simulink model "akh_rev_project"  (R2020b)
settings: Solver=ode45  StartTime=0.0  StopTime=10  FixedStep=Ts_Power  RelTol=1e-3  AbsTol=1e-2
InitFcn:
  | Fnom = 50;        % Hz
  | 
  | Fc = 27*Fnom;   % (Hz)
  | Ts_Power = 1/(Fc*100);
  | Ts_Control = Ts_Power*10;
values from neighbouring files (symbols this model uses):
  Ts = 1/fs    (= 1e-05)    [PE_46.m]    (also in disc_sim.m = 1; mass_spring_damper_model.m = 0.1)
undefined symbols (not defined in the file or in its folder): D1, D11, Delta, DiscIntNeverNeededParam, j, magnitude
libraries: powerlib x146, powerlib_meascontrol x90, simulink x2, re_lib x1
(part 5 of 8)

== system akh_rev_project/AC System 1/Wind Turbine Protection/Protection System/AC Current Protection ==
  abc : Inport  PortDimensions=3
  Complex to Magnitude-Angle1 : ComplexToMagnitudeAngle  Output=Magnitude
  Current Measurement : Subsystem
  MinMax : MinMax  Function=max  InputSameDT=on  SaturateOnIntegerOverflow=on  ZeroCross=off
  Mux : Mux  Inputs=3
  On Delay : powerlib_meascontrol/Logic/On Delay  DelayType=On delay  delay=Delay_I1  ic=0  Ts=0
  On Delay1 : powerlib_meascontrol/Logic/On Delay  DelayType=On delay  delay=Delay_I2_I1  ic=0  Ts=0
  Relational Operator10 : RelationalOperator  Operator=>  RndMeth=Nearest
  Relational Operator6 : RelationalOperator  Operator=>  RndMeth=Nearest
  Relational Operator8 : RelationalOperator  Operator=>  RndMeth=Nearest
  Selector : Selector  InputPortWidth=3  IndexOptions=Index vector (dialog)  Indices=1  OutputSizes=1
  Selector1 : Selector  InputPortWidth=3  IndexOptions=Index vector (dialog)  Indices=2  OutputSizes=1
  Selector2 : Selector  InputPortWidth=3  IndexOptions=Index vector (dialog)  Indices=3  OutputSizes=1
  V0/V1 max3 : Constant  Value=Max_I1
  V1 max : Constant  Value=Max_I2_I1
  V1 max2 : Constant  Value=Max_Iinst
  MaxIinst : Outport  VectorParamsAs1DForOutWhenUnconnected=off
  MaxI1 : Outport  Port=2  VectorParamsAs1DForOutWhenUnconnected=off
  MaxI2I1 : Outport  Port=3  VectorParamsAs1DForOutWhenUnconnected=off
  wires:
  abc/1 -> Current Measurement/1(abc), Selector/1, Selector1/1, Selector2/1
  Current Measurement/1(I1) -> Relational Operator6/1
  V0/V1 max3/1 -> Relational Operator6/2
  V1 max/1 -> Relational Operator8/2
  Current Measurement/2(I2/I1) -> Relational Operator8/1
  Relational Operator6/1 -> On Delay/1
  Relational Operator8/1 -> On Delay1/1
  On Delay/1 -> MaxI1/1
  On Delay1/1 -> MaxI2I1/1
  Relational Operator10/1 -> MaxIinst/1
  V1 max2/1 -> Relational Operator10/2
  Selector/1 -> Mux/1
  Selector2/1 -> Mux/3
  Selector1/1 -> Mux/2
  Mux/1 -> Complex to Magnitude-Angle1/1
  Complex to Magnitude-Angle1/1 -> MinMax/1
  MinMax/1 -> Relational Operator10/1

== system akh_rev_project/AC System 1/Wind Turbine Protection/Protection System/AC Voltage Protection ==
  abc : Inport  PortDimensions=3
  On Delay : powerlib_meascontrol/Logic/On Delay  DelayType=On delay  delay=Delay_V1  ic=0  Ts=0
  On Delay1 : powerlib_meascontrol/Logic/On Delay  DelayType=On delay  delay=Delay_V2_V1  ic=0  Ts=0
  On Delay2 : powerlib_meascontrol/Logic/On Delay  DelayType=On delay  delay=Delay_V1  ic=0  Ts=0
  On Delay3 : powerlib_meascontrol/Logic/On Delay  DelayType=On delay  delay=Delay_V2_V1  ic=0  Ts=0
  Relational Operator6 : RelationalOperator  Operator=>  RndMeth=Nearest
  Relational Operator7 : RelationalOperator  Operator=<  RndMeth=Nearest
  Relational Operator8 : RelationalOperator  Operator=>  RndMeth=Nearest
  Relational Operator9 : RelationalOperator  Operator=>  RndMeth=Nearest
  V0/V1 max3 : Constant  Value=Max_V1
  V0/V1 max4 : Constant  Value=Min_V1
  V1 max : Constant  Value=Max_V2_V1
  V1 max1 : Constant  Value=Max_V0_V1
  Voltage Measurement : Subsystem
  MinV1 : Outport  VectorParamsAs1DForOutWhenUnconnected=off
  MaxV1 : Outport  Port=2  VectorParamsAs1DForOutWhenUnconnected=off
  MaxV2V1 : Outport  Port=3  VectorParamsAs1DForOutWhenUnconnected=off
  MaxV0V1 : Outport  Port=4  VectorParamsAs1DForOutWhenUnconnected=off
  wires:
  On Delay3/1 -> MaxV0V1/1
  On Delay1/1 -> MaxV2V1/1
  On Delay/1 -> MinV1/1
  On Delay2/1 -> MaxV1/1
  Relational Operator9/1 -> On Delay3/1
  Relational Operator8/1 -> On Delay1/1
  Relational Operator7/1 -> On Delay/1
  Relational Operator6/1 -> On Delay2/1
  Voltage Measurement/3(V0/V1) -> Relational Operator9/1
  V1 max1/1 -> Relational Operator9/2
  Voltage Measurement/2(V2/V1) -> Relational Operator8/1
  V1 max/1 -> Relational Operator8/2
  V0/V1 max4/1 -> Relational Operator7/2
  V0/V1 max3/1 -> Relational Operator6/2
  Voltage Measurement/1(V1) -> Relational Operator7/1, Relational Operator6/1
  abc/1 -> Voltage Measurement/1(abc)

== system akh_rev_project/AC System 1/Wind Turbine Protection/Protection System/DC Voltage Protection ==
  Vdc : Inport
  On Delay : powerlib_meascontrol/Logic/On Delay  DelayType=On delay  delay=Delay_Vdc  ic=0  Ts=0
  Relational Operator1 : RelationalOperator  Operator=>  RndMeth=Nearest
  V1 max3 : Constant  Value=Max_Vdc
  MaxVdc : Outport  VectorParamsAs1DForOutWhenUnconnected=off
  wires:
  Vdc/1 -> Relational Operator1/1
  V1 max3/1 -> Relational Operator1/2
  Relational Operator1/1 -> On Delay/1
  On Delay/1 -> MaxVdc/1

== system akh_rev_project/AC System 1/Wind Turbine Protection/Protection System/Decoding ==
  Code : Inport
  Constant : Constant  Value=pow2(0:-1:-9)
  Constant6 : Constant  Value=2
  Math Function : Math  Operator=rem  SignedPower=on  SaturateOnIntegerOverflow=on
  Product : Product  InputSameDT=on  SaturateOnIntegerOverflow=on  OutDataTypeStr=Inherit: Same as first input
  Rounding Function : Rounding
  Out : Outport  VectorParamsAs1DForOutWhenUnconnected=off
  wires:
  Constant/1 -> Product/2
  Code/1 -> Product/1
  Product/1 -> Rounding Function/1
  Constant6/1 -> Math Function/2
  Rounding Function/1 -> Math Function/1
  Math Function/1 -> Out/1

== system akh_rev_project/AC System 1/Wind Turbine Protection/Protection System/Encoding ==
  In1 : Inport
  In2 : Inport  Port=2
  In3 : Inport  Port=3
  In4 : Inport  Port=4
  In5 : Inport  Port=5
  In6 : Inport  Port=6
  In7 : Inport  Port=7
  In8 : Inport  Port=8
  In9 : Inport  Port=9
  In10 : Inport  Port=10
  Constant12 : Constant  Value=pow2(0:1:9)
  Data Type Conversion : DataTypeConversion  SaturateOnIntegerOverflow=on  RndMeth=Zero
  Mux : Mux  Inputs=10
  Product : Product  InputSameDT=on  SaturateOnIntegerOverflow=on  OutDataTypeStr=Inherit: Same as first input
  Sum : Sum  Inputs=1  InputSameDT=on  SaturateOnIntegerOverflow=on  OutDataTypeStr=Inherit: Same as first input
  Code : Outport  VectorParamsAs1DForOutWhenUnconnected=off
  wires:
  Data Type Conversion/1 -> Product/1
  Mux/1 -> Data Type Conversion/1
  In2/1 -> Mux/2
  In3/1 -> Mux/3
  In4/1 -> Mux/4
  In5/1 -> Mux/5
  In6/1 -> Mux/6
  In7/1 -> Mux/7
  In8/1 -> Mux/8
  In9/1 -> Mux/9
  In10/1 -> Mux/10
  In1/1 -> Mux/1
  Product/1 -> Sum/1
  Constant12/1 -> Product/2
  Sum/1 -> Code/1

== system akh_rev_project/AC System 1/Wind Turbine Protection/Protection System/Sample & Hold ==
  note: Silvano Casoria
      | Power System Simulation Laboratory
      | IREQ, Hydro-Quebc
  note: Sample and Hold
  In : Inport
  S : Inport  Port=2
  IC=ic : Memory  InitialCondition=ic  InheritSampleTime=on
  Switch : Switch  Threshold=0.5  SaturateOnIntegerOverflow=on  InputSameDT=on
  "   " : Outport  InitialOutput=0  VectorParamsAs1DForOutWhenUnconnected=off
  wires:
  S/1 -> Switch/2
  In/1 -> Switch/1
  IC=ic/1 -> Switch/3
  Switch/1 -> IC=ic/1, "   "/1

== system akh_rev_project/AC System 1/Wind Turbine Protection/Protection System/Sample & Hold1 ==
  note: Silvano Casoria
      | Power System Simulation Laboratory
      | IREQ, Hydro-Quebc
  note: Sample and Hold
  In : Inport
  S : Inport  Port=2
  IC=ic : Memory  InitialCondition=ic  InheritSampleTime=on
  Switch : Switch  Threshold=0.5  SaturateOnIntegerOverflow=on  InputSameDT=on
  "   " : Outport  InitialOutput=0  VectorParamsAs1DForOutWhenUnconnected=off
  wires:
  S/1 -> Switch/2
  In/1 -> Switch/1
  IC=ic/1 -> Switch/3
  Switch/1 -> IC=ic/1, "   "/1

== system akh_rev_project/AC System 1/Wind Turbine Protection/Protection System/Under//Over Speed Protection ==
  Speed : Inport  PortDimensions=1
  On Delay : powerlib_meascontrol/Logic/On Delay  DelayType=On delay  delay=Delay_Speed  ic=0  Ts=0
  On Delay1 : powerlib_meascontrol/Logic/On Delay  DelayType=On delay  delay=Delay_Speed  ic=0  Ts=0
  Relational Operator1 : RelationalOperator  Operator=>  RndMeth=Nearest
  Relational Operator3 : RelationalOperator  Operator=<  RndMeth=Nearest
  V1 max1 : Constant  Value=Min_Speed
  V1 max3 : Constant  Value=Max_Speed
  MinSpeed : Outport  VectorParamsAs1DForOutWhenUnconnected=off
  MaxSpeed : Outport  Port=2  VectorParamsAs1DForOutWhenUnconnected=off
  wires:
  Relational Operator3/1 -> On Delay/1
  Relational Operator1/1 -> On Delay1/1
  V1 max1/1 -> Relational Operator3/2
  V1 max3/1 -> Relational Operator1/2
  Speed/1 -> Relational Operator3/1, Relational Operator1/1
  On Delay/1 -> MinSpeed/1
  On Delay1/1 -> MaxSpeed/1

== system akh_rev_project/VSC Controller Station 1/Discrete VSC Controller /Clark Transformations/CLARK  with Rotating reference ==
  note: Rotation of pi/6
  note: Rotation of - pi/6
  note: Reference rotation:
      | Type [0,1,2]          Rotation (rad)
      | 0                            0
      | 1                            - pi/6
      | 2                              pi/6
  note: CLARK transformations
  abc : Inport
  Type : Inport  Port=2
  CLARK : Subsystem  TreatAsAtomicUnit=on
  CLARK_lag : Subsystem  TreatAsAtomicUnit=on
  CLARK_lead : Subsystem  TreatAsAtomicUnit=on
  Constant : Constant  Value=2
  Constant1 : Constant  Value=0
  Constant2 : Constant
  Relational Operator1 : RelationalOperator  Operator===  RndMeth=Nearest  InputSameDT=on
  Relational Operator2 : RelationalOperator  Operator===  RndMeth=Nearest  InputSameDT=on
  Relational Operator3 : RelationalOperator  Operator===  RndMeth=Nearest  InputSameDT=on
  Sum : Sum  Inputs=+++  SaturateOnIntegerOverflow=on
  AB0 : Outport  VectorParamsAs1DForOutWhenUnconnected=off
  wires:
  Constant2/1 -> Relational Operator3/2
  Relational Operator2/1 -> CLARK/Enable
  Constant1/1 -> Relational Operator2/2
  CLARK/1(AB0) -> Sum/3
  Sum/1 -> AB0/1
  CLARK_lag/1(AB0) -> Sum/2
  CLARK_lead/1(AB0) -> Sum/1
  abc/1 -> CLARK/1(abc), CLARK_lag/1(abc), CLARK_lead/1(abc)
  Relational Operator1/1 -> CLARK_lead/Enable
  Relational Operator3/1 -> CLARK_lag/Enable
  Type/1 -> Relational Operator3/1, Relational Operator2/1, Relational Operator1/1
  Constant/1 -> Relational Operator1/2

== system akh_rev_project/VSC Controller Station 1/Discrete VSC Controller /Clark Transformations/CLARK  with Rotating reference1 ==
  note: Rotation of pi/6
  note: Rotation of - pi/6
  note: Reference rotation:
      | Type [0,1,2]          Rotation (rad)
      | 0                            0
      | 1                            - pi/6
      | 2                              pi/6
  note: CLARK transformations
  abc : Inport
  Type : Inport  Port=2
  CLARK : Subsystem  TreatAsAtomicUnit=on
  CLARK_lag : Subsystem  TreatAsAtomicUnit=on
  CLARK_lead : Subsystem  TreatAsAtomicUnit=on
  Constant : Constant  Value=2
  Constant1 : Constant  Value=0
  Constant2 : Constant
  Relational Operator1 : RelationalOperator  Operator===  RndMeth=Nearest  InputSameDT=on
  Relational Operator2 : RelationalOperator  Operator===  RndMeth=Nearest  InputSameDT=on
  Relational Operator3 : RelationalOperator  Operator===  RndMeth=Nearest  InputSameDT=on
  Sum : Sum  Inputs=+++  SaturateOnIntegerOverflow=on
  AB0 : Outport  VectorParamsAs1DForOutWhenUnconnected=off
  wires:
  Constant2/1 -> Relational Operator3/2
  Relational Operator2/1 -> CLARK/Enable
  Constant1/1 -> Relational Operator2/2
  CLARK/1(AB0) -> Sum/3
  Sum/1 -> AB0/1
  CLARK_lag/1(AB0) -> Sum/2
  CLARK_lead/1(AB0) -> Sum/1
  abc/1 -> CLARK/1(abc), CLARK_lag/1(abc), CLARK_lead/1(abc)
  Relational Operator1/1 -> CLARK_lead/Enable
  Relational Operator3/1 -> CLARK_lag/Enable
  Type/1 -> Relational Operator3/1, Relational Operator2/1, Relational Operator1/1
  Constant/1 -> Relational Operator1/2

== system akh_rev_project/VSC Controller Station 1/Discrete VSC Controller /DC Voltage Balance Control/Regulator ==
  note: Reset states when enabling
  note: Voltage Sign
  note: Reversed Current Sign
  V_ref_lim_abc : Inport
  Iv_abc : Inport  Port=2
  Udc_0_mean : Inport  Port=3
  Enable : EnablePort  StatesWhenEnabling=reset  PropagateVarSize=During execution
  Constant1 : Constant  Value=0
  Constant2 : Constant  Value=0
  Constant3 : Constant  Value=-1
  Constant4 : Constant
  Constant5 : Constant
  Constant6 : Constant  Value=-1
  Constant7 : Constant  Value=0
  PI_regulator (type 2) : Subsystem  mask(PI regulator with anti-windup - type 2){max_i=max_out_dcvbc, min_i=min_out_dcvbc, Ki=Ki_dcvbc, i_ic=0, Kp=Kp_dcvbc, Kf=1.0, max_out=max_out_dcvbc, min_out=min_out_dcvbc, Ts=Ts_Control}
      mask prompts: max_i "Integrator maximum  limit (pu):"; min_i "Integrator minimum  limit (pu):"; Ki "Integrator gain (pu/s):"; i_ic "Integrator initial condition (pu):"; Kp "Proportional gain:"; Kf "Feadback gain :"; max_out "Output maximum limit (pu):"; min_out "Output minimum limit (pu):"; Ts "Sample time: (s)"
      mask help:
      | The error signal (input 1 - input 2) is integrated with dynamic limits (Integrator min and max limits).
      | A back-calculation anti-windup method discharges the integrator on block saturation (output min and max limits) using a feedback loop having a gain coefficient.
      mask Display: disp('PI \n(Type 2)')
  Product : Product  Inputs=3  SaturateOnIntegerOverflow=on  OutDataTypeStr=Inherit: Same as first input
  Relational Operator : RelationalOperator  Operator=<  RndMeth=Nearest
  Relational Operator1 : RelationalOperator  Operator=<  RndMeth=Nearest
  Switch : Switch  Criteria=u2 > Threshold  SaturateOnIntegerOverflow=on
  Switch1 : Switch  Criteria=u2 > Threshold  SaturateOnIntegerOverflow=on
  dV_ref_abc_dcvbc : Outport  VectorParamsAs1DForOutWhenUnconnected=off
  wires:
  Constant1/1 -> PI_regulator (type 2)/2(Meas)
  Switch1/1 -> Product/2
  PI_regulator (type 2)/1(Out) -> Product/3
  Constant2/1 -> Relational Operator/2
  Constant3/1 -> Switch/1
  Constant4/1 -> Switch/3
  Relational Operator/1 -> Switch/2
  Constant5/1 -> Switch1/1
  Constant6/1 -> Switch1/3
  Relational Operator1/1 -> Switch1/2
  Switch/1 -> Product/1
  V_ref_lim_abc/1 -> Relational Operator/1
  Product/1 -> dV_ref_abc_dcvbc/1
  Iv_abc/1 -> Relational Operator1/1
  Udc_0_mean/1 -> PI_regulator (type 2)/1(Ord)
  Constant7/1 -> Relational Operator1/2

== system akh_rev_project/VSC Controller Station 1/Discrete VSC Controller /Inner Current Loop/AC_Current_Control ==
  note: Gain equal to the converter series reactance in pu
      | (ex: X transformer + X phase reactor)
  note: Uq
  note: Ud
  note: AC Current Control
  note: d axis
  note: q axis
  Iv_dq : Inport
  Iref_dq : Inport  Port=2
  U_dq : Inport  Port=3
  Freq : Inport  Port=4
  Demux : Demux  Outputs=2
      settings: DisplayOption=none
  Demux1 : Demux  Outputs=2
      settings: DisplayOption=none
  Demux2 : Demux  Outputs=2
      settings: DisplayOption=none
  Gain : Gain  Gain=Kf_accc
  Gain1 : Gain  Gain=Kf_accc
  "Mean (Variable Frequency, IC=1)" : powerlib_meascontrol/Measurements/Mean (Variable Frequency)  Finit=Fnom  Fmin=f_min_pll  Vinit=1.0  Ts=Ts_Control
      settings: SourceProductBaseCode=PS
  "Mean (Variable Frequency, IC=1)  " : powerlib_meascontrol/Measurements/Mean (Variable Frequency)  Finit=Fnom  Fmin=f_min_pll  Vinit=1.0  Ts=Ts_Control
      settings: SourceProductBaseCode=PS
  Mux : Mux  Inputs=2
  PI_regulator 1 : Subsystem  mask(PI regulator with anti-windup - type 2){max_i=max_out_accc, min_i=min_out_accc, Ki=Ki_accc, i_ic=0, Kp=Kp_accc, Kf=1.0, max_out=max_out_accc, min_out=min_out_accc, Ts=Ts_Control}
      mask prompts: max_i "Integrator maximum  limit (pu):"; min_i "Integrator minimum  limit (pu):"; Ki "Integrator gain (pu/s):"; i_ic "Integrator initial condition (pu):"; Kp "Proportional gain:"; Kf "Feadback gain :"; max_out "Output maximum limit (pu):"; min_out "Output minimum limit (pu):"; Ts "Sample time: (s)"
      mask help:
      | The error signal (input 1 - input 2) is integrated with dynamic limits (Integrator min and max limits).
      | A back-calculation anti-windup method discharges the integrator on block saturation (output min and max limits) using a feedback loop having a gain coefficient.
      mask Display: disp('PI \n(Type 2)')
  PI_regulator 2 : Subsystem  mask(PI regulator with anti-windup - type 2){max_i=max_out_accc, min_i=min_out_accc, Ki=Ki_accc, i_ic=0, Kp=Kp_accc, Kf=1.0, max_out=max_out_accc, min_out=min_out_accc, Ts=Ts_Control}
      mask prompts: max_i "Integrator maximum  limit (pu):"; min_i "Integrator minimum  limit (pu):"; Ki "Integrator gain (pu/s):"; i_ic "Integrator initial condition (pu):"; Kp "Proportional gain:"; Kf "Feadback gain :"; max_out "Output maximum limit (pu):"; min_out "Output minimum limit (pu):"; Ts "Sample time: (s)"
      mask help:
      | The error signal (input 1 - input 2) is integrated with dynamic limits (Integrator min and max limits).
      | A back-calculation anti-windup method discharges the integrator on block saturation (output min and max limits) using a feedback loop having a gain coefficient.
      mask Display: disp('PI \n(Type 2)')
  Sum2 : Sum  Inputs=+|-|+  InputSameDT=on  SaturateOnIntegerOverflow=on  OutDataTypeStr=Inherit: Same as first input
  Sum3 : Sum  Inputs=--+  InputSameDT=on  SaturateOnIntegerOverflow=on  OutDataTypeStr=Inherit: Same as first input
  Vref_dq_tmp : Outport  VectorParamsAs1DForOutWhenUnconnected=off
  wires:
  PI_regulator 2/1(Out) -> Sum3/1
  Sum3/1 -> Mux/2
  "Mean (Variable Frequency, IC=1)  "/1 -> Sum3/3
  Demux2/2 -> "Mean (Variable Frequency, IC=1)  "/2
  Gain1/1 -> Sum3/2
  Sum2/1 -> Mux/1
  "Mean (Variable Frequency, IC=1)"/1 -> Sum2/1
  Freq/1 -> "Mean (Variable Frequency, IC=1)"/1, "Mean (Variable Frequency, IC=1)  "/1
  Demux2/1 -> "Mean (Variable Frequency, IC=1)"/2
  PI_regulator 1/1(Out) -> Sum2/2
  Iref_dq/1 -> Demux1/1
  Iv_dq/1 -> Demux/1
  Demux1/1 -> PI_regulator 1/1(Ord), Gain1/1  "I_ref_d"
  Demux/1 -> PI_regulator 1/2(Meas)  "Iv_d"
  Demux/2 -> PI_regulator 2/2(Meas)  "Iv_q"
  Mux/1 -> Vref_dq_tmp/1
  U_dq/1 -> Demux2/1
  Demux1/2 -> PI_regulator 2/1(Ord), Gain/1  "I_ref_q"
  Gain/1 -> Sum2/3

== system akh_rev_project/VSC Controller Station 1/Discrete VSC Controller /Inner Current Loop/Reference_Voltage_Conditioning ==
  note: Maximum AC Voltage / DC Voltage (pole-neutral)
  note: Voltage Reference Conditioning
  Vref_dq_tmp : Inport
  Udc_meas_mean : Inport  Port=2
  Constant2 : Constant  Value=K_pwm
  Gain1 : Gain  Gain=k_pu2nom_Vdc  SaturateOnIntegerOverflow=on  OutDataTypeStr=Inherit: Same as input  ParamDataTypeStr=Inherit: Same as input
  Product1 : Product  Inputs=**/  SaturateOnIntegerOverflow=on  OutDataTypeStr=Inherit: Same as first input
  Vref_dq : Outport  VectorParamsAs1DForOutWhenUnconnected=off
  wires:
  Gain1/1 -> Product1/2
  Udc_meas_mean/1 -> Gain1/1
  Product1/1 -> Vref_dq/1
  Vref_dq_tmp/1 -> Product1/1
  Constant2/1 -> Product1/3

== system akh_rev_project/VSC Controller Station 1/Discrete VSC Controller /Inner Current Loop/Reference_Voltage_Limitation ==
  note: Limitation on a circle of 1 p.u. radius
  note: Reference Voltage Limitation
  note: Not Limited
  note: Limited
  Vref_dq : Inport
  Constant2 : Constant  Value=1.0
  Math Function : Math  Operator=magnitude^2  SignedPower=on  SaturateOnIntegerOverflow=on
  Math Function1 : Math  Operator=sqrt  SignedPower=on  SaturateOnIntegerOverflow=on
  Max=inf Min=eps : Saturate  UpperLimit=1e6  LowerLimit=1e-6
  Product : Product  Inputs=/*  SaturateOnIntegerOverflow=on  OutDataTypeStr=Inherit: Same as first input
  Relational Operator1 : RelationalOperator  Operator=<  RndMeth=Nearest
  Sum : Sum  Inputs=+  SaturateOnIntegerOverflow=on
  Switch : Switch  Criteria=u2 > Threshold  SaturateOnIntegerOverflow=on
  Vref_lim_dq : Outport  VectorParamsAs1DForOutWhenUnconnected=off
  wires:
  Max=inf Min=eps/1 -> Product/1
  Relational Operator1/1 -> Switch/2
  Math Function1/1 -> Max=inf Min=eps/1, Relational Operator1/1
  Vref_dq/1 -> Math Function/1, Switch/1, Product/2
  Math Function/1 -> Sum/1
  Sum/1 -> Math Function1/1
  Product/1 -> Switch/3
  Switch/1 -> Vref_lim_dq/1
  Constant2/1 -> Relational Operator1/2

== system akh_rev_project/VSC Controller Station 1/Discrete VSC Controller /Outer Active-Reactive Power and Voltage Loop/Active_Power_Control ==
  note: Output is added to the regulator reference
      |  in order to maintain the DC voltage within
      |  minimum and maximum limits
  note: Active Power Control
  enable_control : Inport
  enable_ramp : Inport  Port=2
  Pref : Inport  Port=3
  dPref : Inport  Port=4
  P_meas : Inport  Port=5
  U_meas : Inport  Port=6
  Udc_meas : Inport  Port=7
  Add : Sum
  DC Voltage Control Override : Subsystem  mask(Regulator with override functionality){max_in=Udc_max, min_in=Udc_min, Ki=Ki_apc_vco, Kp=Kp_apc_vco, IC_i=0, max_out_lim=max_apc_vco, min_out_lim=min_apc_vco, Ts=Ts_Control}
      mask prompts: max_in "Input upper range (pu):"; min_in "Input lower range (pu):"; Ki "Integrator gain (pu/s):"; Kp "Proportional gain:"; IC_i "Integrator initial condition (pu):"; max_out_lim "Output maximum limit (pu):"; min_out_lim "Output minimum limit (pu):"; Ts "Sample time: (s)"
      mask Display: disp('Override \nRegulator')
  Freeze_integrator : Subsystem
  Int_regulator (type 1) : Subsystem  mask(Feed forward integral regulator with anti-windup and freeze - type 1){max_i=max_i_apc, min_i=min_i_apc, Ki=Ki_apc, IC_i=0, Kf=1.0, max_out=P_max, min_out=P_min, Ts=Ts_Control}
      mask prompts: max_i "Integrator maximum  limit (pu):"; min_i "Integrator minimum  limit (pu):"; Ki "Integrator gain (pu/s):"; IC_i "Integrator initial condition (pu):"; Kf "Feadback gain :"; max_out "Output maximum limit (pu):"; min_out "Output minimum limit (pu):"; Ts "Sample time: (s)"
      mask help:
      | The reference (input 1) is fed forward to the output. The integrator compensates for any steady-state error between the desired (input 1) and the measured value input 2). The error signal (input 1 - input 2) is integrated with dynamic limits (Integrator min and max limits). The integration can be frozen (stopped) when input 3 is TRUE.
      | A back-calculation anti-windup method discharges the integrator on block saturation (output min and max limits) using a feedback loop having a gain coefficient.
      mask Display: disp('Integral \n(Type 1)')
  Ramping : Subsystem
  Saturation : Saturate  UpperLimit=P_max  LowerLimit=P_min
      settings: AttributesFormatString=Min=%<LowerLimit>\nMax=%<UpperLimit>
  Sum2 : Sum  SaturateOnIntegerOverflow=on
  Pref_apc : Outport  VectorParamsAs1DForOutWhenUnconnected=off
  Pref_ramped : Outport  Port=2  VectorParamsAs1DForOutWhenUnconnected=off
  wires:
  DC Voltage Control Override/1(Out) -> Add/2
  Int_regulator (type 1)/1(Out) -> Add/1
  Freeze_integrator/1(Freeze) -> Int_regulator (type 1)/3(freeze)
  Add/1 -> Saturation/1
  Saturation/1 -> Pref_apc/1
  Udc_meas/1 -> DC Voltage Control Override/1(In)
  U_meas/1 -> Freeze_integrator/1(U_meas)
  enable_ramp/1 -> Ramping/1(enable_ramp)
  Pref/1 -> Ramping/2(Pref)
  P_meas/1 -> Int_regulator (type 1)/2(Meas)
  Sum2/1 -> Pref_ramped/1, Int_regulator (type 1)/1(Ord)
  dPref/1 -> Sum2/2
  Ramping/1(Pref_ramp) -> Sum2/1
  enable_control/1 -> Int_regulator (type 1)/Enable, DC Voltage Control Override/Enable

== system akh_rev_project/VSC Controller Station 1/Discrete VSC Controller /Outer Active-Reactive Power and Voltage Loop/Current_Reference_Calculation ==
  note: Current Reference Calculation
  Pref_apc : Inport
  Qref_rpc : Inport  Port=2
  Uf_meas : Inport  Port=3
  Constant24 : Constant  Value=U_level_crc
  MinMax : MinMax  Function=max  Inputs=2  InputSameDT=on  SaturateOnIntegerOverflow=on
  Product : Product  Inputs=*/  SaturateOnIntegerOverflow=on  OutDataTypeStr=Inherit: Same as first input
  Product1 : Product  Inputs=/*  SaturateOnIntegerOverflow=on  OutDataTypeStr=Inherit: Same as first input
  Saturation : Saturate  UpperLimit=lim_d_crc  LowerLimit=-lim_d_crc
      settings: AttributesFormatString=Min: %<LowerLimit>\nMax: %<UpperLimit>
  Saturation1 : Saturate  UpperLimit=lim_q_crc  LowerLimit=-lim_q_crc
      settings: AttributesFormatString=Min: %<LowerLimit>\nMax: %<UpperLimit>
  Saturation2 : Saturate  UpperLimit=inf  LowerLimit=eps
      settings: AttributesFormatString=Min: %<LowerLimit>\nMax: %<UpperLimit>
  Second-Order LP Filter : powerlib_meascontrol/Filters/Second-Order Filter  FilterType=Lowpass  Fo=f0_crc  Zeta=1/sqrt(2)  Ts=Ts_Control  Initialize=off  Vac_Init="[0,  0,  60]"  Vdc_Init=0  PlotResponse=off  FreqRange=[0, 500, 1]
      settings: AttributesFormatString=Fo: %<Fo>  SourceProductBaseCode=PS
  Iref_d_crc : Outport  VectorParamsAs1DForOutWhenUnconnected=off
  Iref_q_crc : Outport  Port=2  VectorParamsAs1DForOutWhenUnconnected=off
  wires:
  Second-Order LP Filter/1 -> MinMax/2
  Saturation1/1 -> Iref_q_crc/1
  Saturation/1 -> Iref_d_crc/1
  Uf_meas/1 -> Second-Order LP Filter/1
  Constant24/1 -> MinMax/1
  Pref_apc/1 -> Product/1
  Saturation2/1 -> Product/2, Product1/1
  Qref_rpc/1 -> Product1/2
  Product/1 -> Saturation/1
  Product1/1 -> Saturation1/1
  MinMax/1 -> Saturation2/1

== system akh_rev_project/VSC Controller Station 1/Discrete VSC Controller /Outer Active-Reactive Power and Voltage Loop/Current_Reference_Limitation ==
  note: DC Voltage Control mode (Active power priority)
  note: Power Control mode (Equal scaling)
  note: Current Reference Limitation
  Iref_d_tmp : Inport  PortDimensions=1
  Iref_q_tmp : Inport  Port=2  PortDimensions=1
  P_control : Inport  Port=3
  Constant25 : Constant  Value=Iref_max
  Double click here for  info : Subsystem
      mask Display: disp('?')
  Math Function1 : Math  Operator=sqrt  SignedPower=on  SaturateOnIntegerOverflow=on
  Math Function2 : Math  Operator=magnitude^2  SignedPower=on  SaturateOnIntegerOverflow=on
  Math Function3 : Math  Operator=magnitude^2  SignedPower=on  SaturateOnIntegerOverflow=on
  Math Function4 : Math  Operator=magnitude^2  SignedPower=on  SaturateOnIntegerOverflow=on
  Math Function5 : Math  Operator=sqrt  SignedPower=on  SaturateOnIntegerOverflow=on
  Min:eps Max:inf : Saturate  UpperLimit=1e6  LowerLimit=1e-6
  Mux : Mux  Inputs=2
  Mux1 : Mux  Inputs=2
  Product1 : Product  SaturateOnIntegerOverflow=on  OutDataTypeStr=Inherit: Same as first input
  Product2 : Product  Inputs=*/  SaturateOnIntegerOverflow=on  OutDataTypeStr=Inherit: Same as first input
  Relational Operator1 : RelationalOperator  RndMeth=Nearest
  Relational Operator3 : RelationalOperator  RndMeth=Nearest
  Sign : Signum
  Sum : Sum  Inputs=+  SaturateOnIntegerOverflow=on
  Sum2 : Sum  Inputs=-+  SaturateOnIntegerOverflow=on
  Switch1 : Switch  Criteria=u2 > Threshold  SaturateOnIntegerOverflow=on
  Switch2 : Switch  Criteria=u2 > Threshold  SaturateOnIntegerOverflow=on
  Switch3 : Switch  Criteria=u2 > Threshold  SaturateOnIntegerOverflow=on
  Iref_dq : Outport  VectorParamsAs1DForOutWhenUnconnected=off
  wires:
  Sign/1 -> Product1/2
  Math Function5/1 -> Product1/1
  Product1/1 -> Mux1/2
  Sum2/1 -> Math Function5/1
  Math Function4/1 -> Sum2/1
  Math Function3/1 -> Sum2/2
  Mux1/1 -> Switch2/3
  Switch1/1 -> Iref_dq/1
  Switch2/1 -> Switch1/1
  Product2/1 -> Switch2/1
  Min:eps Max:inf/1 -> Product2/2
  Relational Operator1/1 -> Switch1/2
  Constant25/1 -> Relational Operator3/2, Switch3/1, Math Function3/1, Relational Operator1/2
  Math Function1/1 -> Min:eps Max:inf/1, Relational Operator1/1
  Mux/1 -> Product2/1, Math Function2/1, Switch1/3
  Iref_q_tmp/1 -> Sign/1, Mux/2
  Iref_d_tmp/1 -> Relational Operator3/1, Switch3/3, Mux/1
  Sum/1 -> Math Function1/1
  Math Function2/1 -> Sum/1
  P_control/1 -> Switch2/2
  Relational Operator3/1 -> Switch3/2
  Switch3/1 -> Mux1/1, Math Function4/1

== system akh_rev_project/VSC Controller Station 1/Discrete VSC Controller /Outer Active-Reactive Power and Voltage Loop/DC_Voltage_Control ==
  note: DC Voltage Control
  note: Reset integrator when enabling
  Udref : Inport
  Udc_meas : Inport  Port=2
  Enable (Reset) : EnablePort  StatesWhenEnabling=reset  PropagateVarSize=During execution
  PI_regulator (type 2) : Subsystem  mask(PI regulator with anti-windup - type 2){max_i=max_i_dcvc, min_i=min_i_dcvc, Ki=Ki_dcvc, i_ic=0, Kp=Kp_dcvc, Kf=1.0, max_out=max_out_dcvc, min_out=min_out_dcvc, Ts=Ts_Control}
      mask prompts: max_i "Integrator maximum  limit (pu):"; min_i "Integrator minimum  limit (pu):"; Ki "Integrator gain (pu/s):"; i_ic "Integrator initial condition (pu):"; Kp "Proportional gain:"; Kf "Feadback gain :"; max_out "Output maximum limit (pu):"; min_out "Output minimum limit (pu):"; Ts "Sample time: (s)"
      mask help:
      | The error signal (input 1 - input 2) is integrated with dynamic limits (Integrator min and max limits).
      | A back-calculation anti-windup method discharges the integrator on block saturation (output min and max limits) using a feedback loop having a gain coefficient.
      mask Display: disp('PI \n(Type 2)')
  Iref_d_dcvc : Outport  VectorParamsAs1DForOutWhenUnconnected=off
  wires:
  PI_regulator (type 2)/1(Out) -> Iref_d_dcvc/1
  Udref/1 -> PI_regulator (type 2)/1(Ord)
  Udc_meas/1 -> PI_regulator (type 2)/2(Meas)

== system akh_rev_project/VSC Controller Station 1/Discrete VSC Controller /Outer Active-Reactive Power and Voltage Loop/Reactive_Power_Control ==
  note: Output is added to the regulator reference
      |  in order to maintain the AC voltage within
      |  minimum and maximum limits
  note: Reactive Power Control
  enable_control : Inport
  Qref : Inport  Port=2
  Q_meas : Inport  Port=3
  U_meas : Inport  Port=4
  "AC Voltage Control Override " : Subsystem  mask(Regulator with override functionality){max_in=U_max, min_in=U_min, Ki=Ki_rpc_vco, Kp=Kp_rpc_vco, IC_i=0, max_out_lim=max_rpc_vco, min_out_lim=min_rpc_vco, Ts=Ts_Control}
      mask prompts: max_in "Input upper range (pu):"; min_in "Input lower range (pu):"; Ki "Integrator gain (pu/s):"; Kp "Proportional gain:"; IC_i "Integrator initial condition (pu):"; max_out_lim "Output maximum limit (pu):"; min_out_lim "Output minimum limit (pu):"; Ts "Sample time: (s)"
      mask Display: disp('Override \nRegulator')
  Add : Sum
  Freeze_integrator : Subsystem
  Gain : Gain  Gain=-1
  Int_regulator (type 1) : Subsystem  mask(Feed forward integral regulator with anti-windup and freeze - type 1){max_i=max_i_rpc, min_i=min_i_rpc, Ki=Ki_rpc, IC_i=0, Kf=1.0, max_out=Q_max, min_out=Q_min, Ts=Ts_Control}
      mask prompts: max_i "Integrator maximum  limit (pu):"; min_i "Integrator minimum  limit (pu):"; Ki "Integrator gain (pu/s):"; IC_i "Integrator initial condition (pu):"; Kf "Feadback gain :"; max_out "Output maximum limit (pu):"; min_out "Output minimum limit (pu):"; Ts "Sample time: (s)"
      mask help:
      | The reference (input 1) is fed forward to the output. The integrator compensates for any steady-state error between the desired (input 1) and the measured value input 2). The error signal (input 1 - input 2) is integrated with dynamic limits (Integrator min and max limits). The integration can be frozen (stopped) when input 3 is TRUE.
      | A back-calculation anti-windup method discharges the integrator on block saturation (output min and max limits) using a feedback loop having a gain coefficient.
      mask Display: disp('Integral \n(Type 1)')
  Saturation : Saturate  UpperLimit=Q_max  LowerLimit=Q_min
      settings: AttributesFormatString=Min=%<LowerLimit>\nMax=%<UpperLimit>
  Qref_rpc : Outport  VectorParamsAs1DForOutWhenUnconnected=off
  wires:
  Gain/1 -> Add/1
  Add/1 -> Saturation/1
  "AC Voltage Control Override "/1(Out) -> Add/2
  Int_regulator (type 1)/1(Out) -> Gain/1
  U_meas/1 -> Freeze_integrator/1(U_meas), "AC Voltage Control Override "/1(In)
  Saturation/1 -> Qref_rpc/1
  Qref/1 -> Int_regulator (type 1)/1(Ord)
  Q_meas/1 -> Int_regulator (type 1)/2(Meas)
  enable_control/1 -> Int_regulator (type 1)/Enable, "AC Voltage Control Override "/Enable
  Freeze_integrator/1(Freeze) -> Int_regulator (type 1)/3(freeze)

== system akh_rev_project/VSC Controller Station 1/Discrete VSC Controller /PLL/Discrete PI Controller ==
  note: Pierre Giroux, Gilbert Sybille
      | Power System Simulation Laboratory
      | IREQ, Hydro-Quebc
  note: Discrete PID Controller
  Error : Inport  SampleTime=Ts
  Discrete-Time Integrator : DiscreteIntegrator  InitialCondition=Init  SampleTime=Ts  LimitOutput=on  UpperSaturationLimit=UpperLimit  LowerSaturationLimit=LowerLimit  ICPrevOutput=DiscIntNeverNeededParam  ICPrevScaledInput=DiscIntNeverNeededParam
  Kp4 : Gain  Gain=Kp  SaturateOnIntegerOverflow=on  SampleTime=Ts  OutDataTypeStr=Inherit: Same as input  ParamDataTypeStr=Inherit: Same as input
  Kp5 : Gain  Gain=Ki  SaturateOnIntegerOverflow=on  SampleTime=Ts  OutDataTypeStr=Inherit: Same as input  ParamDataTypeStr=Inherit: Same as input
  Saturation2 : Saturate  UpperLimit=UpperLimit  LowerLimit=LowerLimit  SampleTime=Ts
  Sum6 : Sum  InputSameDT=on  SaturateOnIntegerOverflow=on  SampleTime=Ts  OutDataTypeStr=Inherit: Same as first input
  Zero-Order Hold : ZeroOrderHold  SampleTime=Ts
  Out : Outport  SampleTime=Ts  InitialOutput=0  VectorParamsAs1DForOutWhenUnconnected=off
  wires:
  Error/1 -> Kp4/1, Kp5/1
  Sum6/1 -> Saturation2/1
  Kp5/1 -> Discrete-Time Integrator/1
  Kp4/1 -> Zero-Order Hold/1
  Discrete-Time Integrator/1 -> Sum6/2
  Saturation2/1 -> Out/1
  Zero-Order Hold/1 -> Sum6/1

== system akh_rev_project/VSC Controller Station 1/Discrete VSC Controller /PLL/Discrete Rate Limiter ==
  note: Delta(u)
  note: Beat Ronner
      | ABB Industrie AG
      | Turgi, Switzerland
  In : Inport
  Saturation : Saturate  UpperLimit=UpperLimit  LowerLimit=LowerLimit
  Sum : Sum  Inputs=|++  InputSameDT=on  SaturateOnIntegerOverflow=on  OutDataTypeStr=Inherit: Same as first input
  Sum1 : Sum  Inputs=|+-  InputSameDT=on  SaturateOnIntegerOverflow=on  OutDataTypeStr=Inherit: Same as first input
  Unit Delay : UnitDelay  InitialCondition=Vinit  SampleTime=Ts  HasFrameUpgradeWarning=on
  Out : Outport  VectorParamsAs1DForOutWhenUnconnected=off
  wires:
  In/1 -> Sum1/1  "u"
  Sum1/1 -> Saturation/1
  Saturation/1 -> Sum/1  "Delta(u)_limit"
  Sum/1 -> Out/1, Unit Delay/1  "y"
  Unit Delay/1 -> Sum1/2, Sum/2  "y-1"

== system akh_rev_project/VSC Controller Station 1/Discrete VSC Controller /Signal Calculations/Active_Power ==
  note: Active Power Calculation
  U_AB : Inport
  I_AB : Inport  Port=2
  Demux : Demux  Outputs=2
      settings: DisplayOption=none
  Demux1 : Demux  Outputs=2
      settings: DisplayOption=none
  Product : Product  SaturateOnIntegerOverflow=on  OutDataTypeStr=Inherit: Same as first input
  Product1 : Product  SaturateOnIntegerOverflow=on  OutDataTypeStr=Inherit: Same as first input
  Sum : Sum  SaturateOnIntegerOverflow=on
  Ppcc : Outport  VectorParamsAs1DForOutWhenUnconnected=off
  wires:
  U_AB/1 -> Demux/1
  I_AB/1 -> Demux1/1
  Demux/1 -> Product/1
  Demux1/1 -> Product/2
  Demux/2 -> Product1/1
  Demux1/2 -> Product1/2
  Product/1 -> Sum/1
  Product1/1 -> Sum/2
  Sum/1 -> Ppcc/1

== system akh_rev_project/VSC Controller Station 1/Discrete VSC Controller /Signal Calculations/DC_Current ==
  note: DC Current Calculation
  Idc_p : Inport
  Idc_n : Inport  Port=2
  Gain : Gain  Gain=0.5  SaturateOnIntegerOverflow=on  OutDataTypeStr=Inherit: Same as input  ParamDataTypeStr=Inherit: Same as input
  Sum : Sum  Inputs=+-  SaturateOnIntegerOverflow=on
  Idc_meas : Outport  VectorParamsAs1DForOutWhenUnconnected=off
  wires:
  Gain/1 -> Idc_meas/1
  Sum/1 -> Gain/1
  Idc_n/1 -> Sum/2
  Idc_p/1 -> Sum/1

== system akh_rev_project/VSC Controller Station 1/Discrete VSC Controller /Signal Calculations/DC_Voltage ==
  note: DC Voltage Calculation
  Udc_p : Inport
  Udc_n : Inport  Port=2
  Gain : Gain  Gain=0.5  SaturateOnIntegerOverflow=on  OutDataTypeStr=Inherit: Same as input  ParamDataTypeStr=Inherit: Same as input
  Sum : Sum  Inputs=+-  SaturateOnIntegerOverflow=on
  Udc_meas : Outport  VectorParamsAs1DForOutWhenUnconnected=off
  wires:
  Udc_p/1 -> Sum/1
  Sum/1 -> Gain/1
  Gain/1 -> Udc_meas/1
  Udc_n/1 -> Sum/2

== system akh_rev_project/VSC Controller Station 1/Discrete VSC Controller /Signal Calculations/Filter_Bus_Voltage ==
  note: Filter Bus Voltage Calculation
  Uf_AB : Inport
  Math Function : Math  Operator=magnitude^2  SignedPower=on  SaturateOnIntegerOverflow=on
  Math Function1 : Math  Operator=sqrt  SignedPower=on  SaturateOnIntegerOverflow=on
  Sum : Sum  Inputs=+  SaturateOnIntegerOverflow=on
  Uf_meas : Outport  VectorParamsAs1DForOutWhenUnconnected=off
  wires:
  Math Function1/1 -> Uf_meas/1
  Sum/1 -> Math Function1/1
  Math Function/1 -> Sum/1
  Uf_AB/1 -> Math Function/1

== system akh_rev_project/VSC Controller Station 1/Discrete VSC Controller /Signal Calculations/Modulation_Index ==
  note: Modulation Index Calculation
  Vref_lim_AB : Inport
  Udc_meas : Inport  Port=2
  Gain1 : Gain  Gain=k_pu2nom_Vdc  SaturateOnIntegerOverflow=on  OutDataTypeStr=Inherit: Same as input  ParamDataTypeStr=Inherit: Same as input
  MAX:10 MIN: 0 : Saturate  UpperLimit=10  LowerLimit=0
  Math Function1 : Math  Operator=magnitude^2  SignedPower=on  SaturateOnIntegerOverflow=on
  Math Function2 : Math  Operator=sqrt  SignedPower=on  SaturateOnIntegerOverflow=on
  Product : Product  Inputs=*/  SaturateOnIntegerOverflow=on  OutDataTypeStr=Inherit: Same as first input
  Saturation : Saturate  UpperLimit=1e6  LowerLimit=1e-6
  Sum : Sum  Inputs=+  SaturateOnIntegerOverflow=on
  Mod_index : Outport  VectorParamsAs1DForOutWhenUnconnected=off
  wires:
  Gain1/1 -> Saturation/1
  MAX:10 MIN: 0/1 -> Mod_index/1
  Saturation/1 -> Product/2
  Product/1 -> MAX:10 MIN: 0/1
  Udc_meas/1 -> Gain1/1
  Sum/1 -> Math Function2/1
  Math Function1/1 -> Sum/1
  Math Function2/1 -> Product/1
  Vref_lim_AB/1 -> Math Function1/1

== system akh_rev_project/VSC Controller Station 1/Discrete VSC Controller /Signal Calculations/PCC_Voltage ==
  note: Active Power Calculation
  U_AB : Inport
  Math Function : Math  Operator=magnitude^2  SignedPower=on  SaturateOnIntegerOverflow=on
  Math Function1 : Math  Operator=sqrt  SignedPower=on  SaturateOnIntegerOverflow=on
  Sum : Sum  Inputs=+  SaturateOnIntegerOverflow=on
  Upcc : Outport  VectorParamsAs1DForOutWhenUnconnected=off
  wires:
  U_AB/1 -> Math Function/1
  Math Function/1 -> Sum/1
  Sum/1 -> Math Function1/1
  Math Function1/1 -> Upcc/1

== system akh_rev_project/VSC Controller Station 1/Discrete VSC Controller /Signal Calculations/Reactive_Power ==
  note: Reactive Power Calculation
  U_AB : Inport
  I_AB : Inport  Port=2
  Demux : Demux  Outputs=2
      settings: DisplayOption=none
  Demux1 : Demux  Outputs=2
      settings: DisplayOption=none
  Product : Product  SaturateOnIntegerOverflow=on  OutDataTypeStr=Inherit: Same as first input
  Product1 : Product  SaturateOnIntegerOverflow=on  OutDataTypeStr=Inherit: Same as first input
  Sum : Sum  Inputs=+-  SaturateOnIntegerOverflow=on
  Qpcc : Outport  VectorParamsAs1DForOutWhenUnconnected=off
  wires:
  Sum/1 -> Qpcc/1
  Product1/1 -> Sum/2
  Product/1 -> Sum/1
  I_AB/1 -> Demux1/1
  U_AB/1 -> Demux/1
  Demux/2 -> Product/2
  Demux1/1 -> Product/1
  Demux/1 -> Product1/1
  Demux1/2 -> Product1/2

== system akh_rev_project/VSC Controller Station 2/Discrete VSC Controller /Clark Transformations/CLARK  with Rotating reference ==
  note: Rotation of pi/6
  note: Rotation of - pi/6
  note: Reference rotation:
      | Type [0,1,2]          Rotation (rad)
      | 0                            0
      | 1                            - pi/6
      | 2                              pi/6
  note: CLARK transformations
  abc : Inport
  Type : Inport  Port=2
  CLARK : Subsystem  TreatAsAtomicUnit=on
  CLARK_lag : Subsystem  TreatAsAtomicUnit=on
  CLARK_lead : Subsystem  TreatAsAtomicUnit=on
  Constant : Constant  Value=2
  Constant1 : Constant  Value=0
  Constant2 : Constant
  Relational Operator1 : RelationalOperator  Operator===  RndMeth=Nearest  InputSameDT=on
  Relational Operator2 : RelationalOperator  Operator===  RndMeth=Nearest  InputSameDT=on
  Relational Operator3 : RelationalOperator  Operator===  RndMeth=Nearest  InputSameDT=on
  Sum : Sum  Inputs=+++  SaturateOnIntegerOverflow=on
  AB0 : Outport  VectorParamsAs1DForOutWhenUnconnected=off
  wires:
  Constant2/1 -> Relational Operator3/2
  Relational Operator2/1 -> CLARK/Enable
  Constant1/1 -> Relational Operator2/2
  CLARK/1(AB0) -> Sum/3
  Sum/1 -> AB0/1
  CLARK_lag/1(AB0) -> Sum/2
  CLARK_lead/1(AB0) -> Sum/1
  abc/1 -> CLARK/1(abc), CLARK_lag/1(abc), CLARK_lead/1(abc)
  Relational Operator1/1 -> CLARK_lead/Enable
  Relational Operator3/1 -> CLARK_lag/Enable
  Type/1 -> Relational Operator3/1, Relational Operator2/1, Relational Operator1/1
  Constant/1 -> Relational Operator1/2

== system akh_rev_project/VSC Controller Station 2/Discrete VSC Controller /Clark Transformations/CLARK  with Rotating reference1 ==
  note: Rotation of pi/6
  note: Rotation of - pi/6
  note: Reference rotation:
      | Type [0,1,2]          Rotation (rad)
      | 0                            0
      | 1                            - pi/6
      | 2                              pi/6
  note: CLARK transformations
  abc : Inport
  Type : Inport  Port=2
  CLARK : Subsystem  TreatAsAtomicUnit=on
  CLARK_lag : Subsystem  TreatAsAtomicUnit=on
  CLARK_lead : Subsystem  TreatAsAtomicUnit=on
  Constant : Constant  Value=2
  Constant1 : Constant  Value=0
  Constant2 : Constant
  Relational Operator1 : RelationalOperator  Operator===  RndMeth=Nearest  InputSameDT=on
  Relational Operator2 : RelationalOperator  Operator===  RndMeth=Nearest  InputSameDT=on
  Relational Operator3 : RelationalOperator  Operator===  RndMeth=Nearest  InputSameDT=on
  Sum : Sum  Inputs=+++  SaturateOnIntegerOverflow=on
  AB0 : Outport  VectorParamsAs1DForOutWhenUnconnected=off
  wires:
  Constant2/1 -> Relational Operator3/2
  Relational Operator2/1 -> CLARK/Enable
  Constant1/1 -> Relational Operator2/2
  CLARK/1(AB0) -> Sum/3
  Sum/1 -> AB0/1
  CLARK_lag/1(AB0) -> Sum/2
  CLARK_lead/1(AB0) -> Sum/1
  abc/1 -> CLARK/1(abc), CLARK_lag/1(abc), CLARK_lead/1(abc)
  Relational Operator1/1 -> CLARK_lead/Enable
  Relational Operator3/1 -> CLARK_lag/Enable
  Type/1 -> Relational Operator3/1, Relational Operator2/1, Relational Operator1/1
  Constant/1 -> Relational Operator1/2

== system akh_rev_project/VSC Controller Station 2/Discrete VSC Controller /DC Voltage Balance Control/Regulator ==
  note: Reset states when enabling
  note: Voltage Sign
  note: Reversed Current Sign
  V_ref_lim_abc : Inport
  Iv_abc : Inport  Port=2
  Udc_0_mean : Inport  Port=3
  Enable : EnablePort  StatesWhenEnabling=reset  PropagateVarSize=During execution
  Constant1 : Constant  Value=0
  Constant2 : Constant  Value=0
  Constant3 : Constant  Value=-1
  Constant4 : Constant
  Constant5 : Constant
  Constant6 : Constant  Value=-1
  Constant7 : Constant  Value=0
  PI_regulator (type 2) : Subsystem  mask(PI regulator with anti-windup - type 2){max_i=max_out_dcvbc, min_i=min_out_dcvbc, Ki=Ki_dcvbc, i_ic=0, Kp=Kp_dcvbc, Kf=1.0, max_out=max_out_dcvbc, min_out=min_out_dcvbc, Ts=Ts_Control}
      mask prompts: max_i "Integrator maximum  limit (pu):"; min_i "Integrator minimum  limit (pu):"; Ki "Integrator gain (pu/s):"; i_ic "Integrator initial condition (pu):"; Kp "Proportional gain:"; Kf "Feadback gain :"; max_out "Output maximum limit (pu):"; min_out "Output minimum limit (pu):"; Ts "Sample time: (s)"
      mask help:
      | The error signal (input 1 - input 2) is integrated with dynamic limits (Integrator min and max limits).
      | A back-calculation anti-windup method discharges the integrator on block saturation (output min and max limits) using a feedback loop having a gain coefficient.
      mask Display: disp('PI \n(Type 2)')
  Product : Product  Inputs=3  SaturateOnIntegerOverflow=on  OutDataTypeStr=Inherit: Same as first input
  Relational Operator : RelationalOperator  Operator=<  RndMeth=Nearest
  Relational Operator1 : RelationalOperator  Operator=<  RndMeth=Nearest
  Switch : Switch  Criteria=u2 > Threshold  SaturateOnIntegerOverflow=on
  Switch1 : Switch  Criteria=u2 > Threshold  SaturateOnIntegerOverflow=on
  dV_ref_abc_dcvbc : Outport  VectorParamsAs1DForOutWhenUnconnected=off
  wires:
  Constant1/1 -> PI_regulator (type 2)/2(Meas)
  Switch1/1 -> Product/2
  PI_regulator (type 2)/1(Out) -> Product/3
  Constant2/1 -> Relational Operator/2
  Constant3/1 -> Switch/1
  Constant4/1 -> Switch/3
  Relational Operator/1 -> Switch/2
  Constant5/1 -> Switch1/1
  Constant6/1 -> Switch1/3
  Relational Operator1/1 -> Switch1/2
  Switch/1 -> Product/1
  V_ref_lim_abc/1 -> Relational Operator/1
  Product/1 -> dV_ref_abc_dcvbc/1
  Iv_abc/1 -> Relational Operator1/1
  Udc_0_mean/1 -> PI_regulator (type 2)/1(Ord)
  Constant7/1 -> Relational Operator1/2

== system akh_rev_project/VSC Controller Station 2/Discrete VSC Controller /Inner Current Loop/AC_Current_Control ==
  note: Gain equal to the converter series reactance in pu
      | (ex: X transformer + X phase reactor)
  note: Uq
  note: Ud
  note: AC Current Control
  note: d axis
  note: q axis
  Iv_dq : Inport
  Iref_dq : Inport  Port=2
  U_dq : Inport  Port=3
  Freq : Inport  Port=4
  Demux : Demux  Outputs=2
      settings: DisplayOption=none
  Demux1 : Demux  Outputs=2
      settings: DisplayOption=none
  Demux2 : Demux  Outputs=2
      settings: DisplayOption=none
  Gain : Gain  Gain=Kf_accc
  Gain1 : Gain  Gain=Kf_accc
  "Mean (Variable Frequency, IC=1)" : powerlib_meascontrol/Measurements/Mean (Variable Frequency)  Finit=Fnom  Fmin=f_min_pll  Vinit=1.0  Ts=Ts_Control
      settings: SourceProductBaseCode=PS
  "Mean (Variable Frequency, IC=1)  " : powerlib_meascontrol/Measurements/Mean (Variable Frequency)  Finit=Fnom  Fmin=f_min_pll  Vinit=1.0  Ts=Ts_Control
      settings: SourceProductBaseCode=PS
  Mux : Mux  Inputs=2
  PI_regulator 1 : Subsystem  mask(PI regulator with anti-windup - type 2){max_i=max_out_accc, min_i=min_out_accc, Ki=Ki_accc, i_ic=0, Kp=Kp_accc, Kf=1.0, max_out=max_out_accc, min_out=min_out_accc, Ts=Ts_Control}
      mask prompts: max_i "Integrator maximum  limit (pu):"; min_i "Integrator minimum  limit (pu):"; Ki "Integrator gain (pu/s):"; i_ic "Integrator initial condition (pu):"; Kp "Proportional gain:"; Kf "Feadback gain :"; max_out "Output maximum limit (pu):"; min_out "Output minimum limit (pu):"; Ts "Sample time: (s)"
      mask help:
      | The error signal (input 1 - input 2) is integrated with dynamic limits (Integrator min and max limits).
      | A back-calculation anti-windup method discharges the integrator on block saturation (output min and max limits) using a feedback loop having a gain coefficient.
      mask Display: disp('PI \n(Type 2)')
  PI_regulator 2 : Subsystem  mask(PI regulator with anti-windup - type 2){max_i=max_out_accc, min_i=min_out_accc, Ki=Ki_accc, i_ic=0, Kp=Kp_accc, Kf=1.0, max_out=max_out_accc, min_out=min_out_accc, Ts=Ts_Control}
      mask prompts: max_i "Integrator maximum  limit (pu):"; min_i "Integrator minimum  limit (pu):"; Ki "Integrator gain (pu/s):"; i_ic "Integrator initial condition (pu):"; Kp "Proportional gain:"; Kf "Feadback gain :"; max_out "Output maximum limit (pu):"; min_out "Output minimum limit (pu):"; Ts "Sample time: (s)"
      mask help:
      | The error signal (input 1 - input 2) is integrated with dynamic limits (Integrator min and max limits).
      | A back-calculation anti-windup method discharges the integrator on block saturation (output min and max limits) using a feedback loop having a gain coefficient.
      mask Display: disp('PI \n(Type 2)')
  Sum2 : Sum  Inputs=+|-|+  InputSameDT=on  SaturateOnIntegerOverflow=on  OutDataTypeStr=Inherit: Same as first input
  Sum3 : Sum  Inputs=--+  InputSameDT=on  SaturateOnIntegerOverflow=on  OutDataTypeStr=Inherit: Same as first input
  Vref_dq_tmp : Outport  VectorParamsAs1DForOutWhenUnconnected=off
  wires:
  PI_regulator 2/1(Out) -> Sum3/1
  Sum3/1 -> Mux/2
  "Mean (Variable Frequency, IC=1)  "/1 -> Sum3/3
  Demux2/2 -> "Mean (Variable Frequency, IC=1)  "/2
  Gain1/1 -> Sum3/2
  Sum2/1 -> Mux/1
  "Mean (Variable Frequency, IC=1)"/1 -> Sum2/1
  Freq/1 -> "Mean (Variable Frequency, IC=1)"/1, "Mean (Variable Frequency, IC=1)  "/1
  Demux2/1 -> "Mean (Variable Frequency, IC=1)"/2
  PI_regulator 1/1(Out) -> Sum2/2
  Iref_dq/1 -> Demux1/1
  Iv_dq/1 -> Demux/1
  Demux1/1 -> PI_regulator 1/1(Ord), Gain1/1  "I_ref_d"
  Demux/1 -> PI_regulator 1/2(Meas)  "Iv_d"
  Demux/2 -> PI_regulator 2/2(Meas)  "Iv_q"
  Mux/1 -> Vref_dq_tmp/1
  U_dq/1 -> Demux2/1
  Demux1/2 -> PI_regulator 2/1(Ord), Gain/1  "I_ref_q"
  Gain/1 -> Sum2/3

== system akh_rev_project/VSC Controller Station 2/Discrete VSC Controller /Inner Current Loop/Reference_Voltage_Conditioning ==
  note: Maximum AC Voltage / DC Voltage (pole-neutral)
  note: Voltage Reference Conditioning
  Vref_dq_tmp : Inport
  Udc_meas_mean : Inport  Port=2
  Constant2 : Constant  Value=K_pwm
  Gain1 : Gain  Gain=k_pu2nom_Vdc  SaturateOnIntegerOverflow=on  OutDataTypeStr=Inherit: Same as input  ParamDataTypeStr=Inherit: Same as input
  Product1 : Product  Inputs=**/  SaturateOnIntegerOverflow=on  OutDataTypeStr=Inherit: Same as first input
  Vref_dq : Outport  VectorParamsAs1DForOutWhenUnconnected=off
  wires:
  Gain1/1 -> Product1/2
  Udc_meas_mean/1 -> Gain1/1
  Product1/1 -> Vref_dq/1
  Vref_dq_tmp/1 -> Product1/1
  Constant2/1 -> Product1/3
